simulink model "step10"  (R2017b)
settings: Solver=VariableStepAuto  StartTime=0.0  StopTime=10.0  RelTol=1e-3
libraries: powerlib x6
settings Model: Creator=aniko  LastModifiedBy=aniko

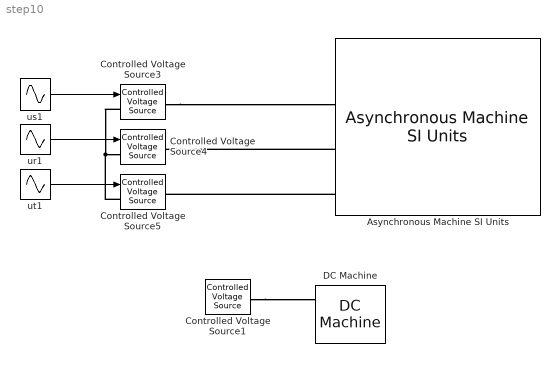
== system step10 ==
  Asynchronous Machine SI Units : powerlib/Machines/Asynchronous Machine SI Units  RotorType=Squirrel-cage  PresetModel=No  MechanicalLoad=Speed w  ShowDetailedParameters=on  ReferenceFrame=Rotor  Units=SI  MeasurementBus=off  NominalParameters=[5500 400 50]  Stator=[0.5968 0.0003495]  Rotor=[0.6258 0.005473]  Cage1=[0.4155 0.002066]  Cage2=[0.4168 0.0003495]  Lm=0.0354  Mechanical=[0.05 0.005879 3]  PolePairs=3  InitialConditions=[0 0 0 0 0 0 0 0]  SimulateSaturation=off  Saturation=[14.03593122, 27.81365428, 53.79336849, 72.68890987, 97.98006896, 148.6815601, 215.7428561, 302.9841135, 428.7778367 ; 230, 322, 414, 460, 506, 552, 598, 644, 690]  LoadFlowParameters=1492000  TsPowergui=0  TsBlock=-1  IterativeModel=Trapezoidal non iterative  IterativeDiscreteModel=Trapezoidal non iterative  Pmec=1.492e+006
  Controlled Voltage Source{1,3..5} (4 alike) : powerlib/Electrical Sources/Controlled Voltage Source  Initialize=on  Source_Type=AC  Amplitude=0  Phase=0  Frequency=0  Measurements=None
  DC Machine : powerlib/Machines/DC Machine  PresetModel=No  MechanicalLoad=Torque TL  FieldType=Permanent magnet  ShowDetailedParameters=on  MeasurementBus=off  RLa=[ 0.1 10e-3]  RLf="[ 240  120]"  Laf=1.8  MachineConstant=Back-emf constant (V/rpm)  Ke=205/1000  Kt=1.8  J=1  Bm=0  Tf=0  w0=1  Ifinit=1  TsPowergui=0  TsBlock=-1
  ur1 : Sin  Amplitude=325  Frequency=50*2*pi  Phase=(-2/3*pi)  SampleTime=0
  us1 : Sin  Amplitude=325  Frequency=50*2*pi  SampleTime=0
  ut1 : Sin  Amplitude=325  Frequency=50*2*pi  Phase=(2/3)*pi  SampleTime=0
  wires:
  us1/1 -> Controlled Voltage Source3/1
  ur1/1 -> Controlled Voltage Source4/1
  ut1/1 -> Controlled Voltage Source5/1
  connections:
  Controlled Voltage Source3/LConn1 -- Controlled Voltage Source5/LConn1 -- Controlled Voltage Source4/LConn1
  Asynchronous Machine SI Units/LConn3 -- Controlled Voltage Source5/RConn1
  Asynchronous Machine SI Units/LConn2 -- Controlled Voltage Source4/RConn1
  Controlled Voltage Source3/RConn1 -- Asynchronous Machine SI Units/LConn1
  Controlled Voltage Source1/RConn1 -- DC Machine/RConn1
